simulink model "doa_no_gotos"  (R2013b)
settings: Solver=ode45  StartTime=0.0  StopTime=10.0  RelTol=1e-3
undefined symbols (not defined in the file or in its folder): calan_lib, comp_addsub
libraries: xbsIndex_r4 x1532, casper_library_misc x168, casper_library_delays x24
(part 2 of 16)

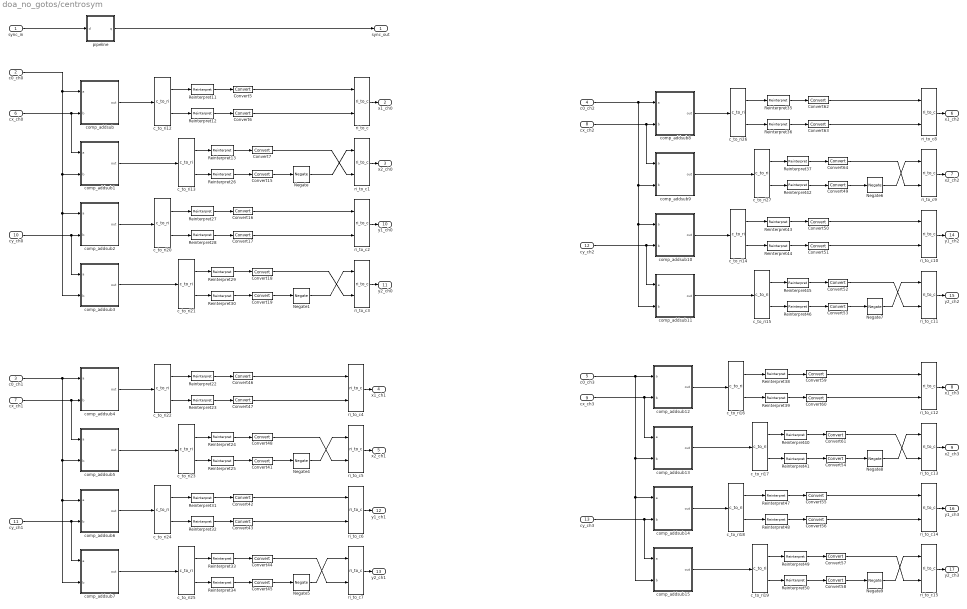
== system doa_no_gotos/centrosym ==
  sync_in : Inport
  c0_ch0 : Inport  Port=2
  c0_ch1 : Inport  Port=3
  c0_ch2 : Inport  Port=4
  c0_ch3 : Inport  Port=5
  cx_ch0 : Inport  Port=6
  cx_ch1 : Inport  Port=7
  cx_ch2 : Inport  Port=8
  cx_ch3 : Inport  Port=9
  cy_ch0 : Inport  Port=10
  cy_ch1 : Inport  Port=11
  cy_ch2 : Inport  Port=12
  cy_ch3 : Inport  Port=13
  Convert{5..7,15..19,41..64} (32 alike) : xbsIndex_r4/Convert  gui_display_data_type=Fixed-point  arith_type="Signed  (2's comp)"  n_bits=8  bin_pt=7  float_type=Single  exp_bits=8  fraction_bits=24  quantization="Round  (unbiased: +/- Inf)"  overflow=Saturate  en=off  latency=0  dbl_ovrd=off  pipeline=off  block_type=convert
  Negate{,1,4..9} (8 alike) : xbsIndex_r4/Negate  precision=User Defined  arith_type="Signed  (2's comp)"  n_bits=8  bin_pt=7  quantization="Round  (unbiased: +/- Inf)"  overflow=Saturate  en=off  latency=0  dbl_ovrd=off  block_type=negate
  Reinterpret{11..13,22..50} (32 alike) : xbsIndex_r4/Reinterpret  force_arith_type=on  arith_type="Signed  (2's comp)"  force_bin_pt=on  bin_pt=8  block_type=reinterpret
  c_to_ri{12..27} (16 alike) : casper_library_misc/c_to_ri  n_bits=9  bin_pt=7
      settings: AttributesFormatString=9_7 r/i
  comp_addsub : Subsystem  AncestorBlock=calan_lib/comp_addsub  mask(comp_addsub){addsub=Addition, n_bits_in=8, bin_pt_in=7, add_latency=2, n_bits_out=9, bin_pt_out=7, quantization=Round  (unbiased: +/- Inf), overflow=Saturate}
      mask prompts: addsub "Addition/Subtraction"; n_bits_in "Bit Width"; bin_pt_in "Binary Point"; add_latency "Adder Latency"; n_bits_out "Bit Width"; bin_pt_out "BInary Point"
      mask help: Add or substract two complex numbers of the same length.
      mask init:
      | comp_addsub_init(gcb, ...
      |     'addsub', addsub, ...
      |     'n_bits_in', n_bits_in, ...
      |     'bin_pt_in', bin_pt_in, ...
      |     'n_bits_out', n_bits_out, ...
      |     'bin_pt_out', bin_pt_out, ...
      |     'quantization', quantization, ...
      |     'overflow', overflow, ...
      |     'add_latency', add_latency);
      settings: AttributesFormatString=|
      | 8_7 * 8_7 ==> 9_7
      | Round  (unbiased: +/- Inf), Saturate
      mask TypeOptions addsub: Addition | Subtraction
      mask TypeOptions quantization: Truncate | Round  (unbiased: +/- Inf)
      mask TypeOptions overflow: Wrap | Saturate | Flag as error
      mask Display:
      | port_label('input', 1, 'a');
      | port_label('input', 2, 'b');
      | if strcmp(addsub, 'Addition')
      |     port_label('output', 1, 'a+b');
      | elseif strcmp(addsub, 'Subtraction')
      |     port_label('output', 1, 'a-b');
      | end
      | disp(['Z^-', num2str(add_latency)]);
  comp_addsub1 : Subsystem  AncestorBlock=calan_lib/comp_addsub  mask(comp_addsub){addsub=Subtraction, n_bits_in=8, bin_pt_in=7, add_latency=2, n_bits_out=9, bin_pt_out=7, quantization=Round  (unbiased: +/- Inf), overflow=Saturate}
      mask prompts: addsub "Addition/Subtraction"; n_bits_in "Bit Width"; bin_pt_in "Binary Point"; add_latency "Adder Latency"; n_bits_out "Bit Width"; bin_pt_out "BInary Point"
      mask help: Add or substract two complex numbers of the same length.
      mask init: same as doa_no_gotos/centrosym/comp_addsub
      settings: AttributesFormatString=|
      | 8_7 * 8_7 ==> 9_7
      | Round  (unbiased: +/- Inf), Saturate
      mask TypeOptions addsub: Addition | Subtraction
      mask TypeOptions quantization: Truncate | Round  (unbiased: +/- Inf)
      mask TypeOptions overflow: Wrap | Saturate | Flag as error
      mask Display:
      | port_label('input', 1, 'a');
      | port_label('input', 2, 'b');
      | if strcmp(addsub, 'Addition')
      |     port_label('output', 1, 'a+b');
      | elseif strcmp(addsub, 'Subtraction')
      |     port_label('output', 1, 'a-b');
      | end
      | disp(['Z^-', num2str(add_latency)]);
  comp_addsub10 : Subsystem  AncestorBlock=calan_lib/comp_addsub  mask(comp_addsub){addsub=Addition, n_bits_in=8, bin_pt_in=7, add_latency=2, n_bits_out=9, bin_pt_out=7, quantization=Round  (unbiased: +/- Inf), overflow=Saturate}
      mask prompts: addsub "Addition/Subtraction"; n_bits_in "Bit Width"; bin_pt_in "Binary Point"; add_latency "Adder Latency"; n_bits_out "Bit Width"; bin_pt_out "BInary Point"
      mask help: Add or substract two complex numbers of the same length.
      mask init: same as doa_no_gotos/centrosym/comp_addsub
      settings: AttributesFormatString=|
      | 8_7 * 8_7 ==> 9_7
      | Round  (unbiased: +/- Inf), Saturate
      mask TypeOptions addsub: Addition | Subtraction
      mask TypeOptions quantization: Truncate | Round  (unbiased: +/- Inf)
      mask TypeOptions overflow: Wrap | Saturate | Flag as error
      mask Display:
      | port_label('input', 1, 'a');
      | port_label('input', 2, 'b');
      | if strcmp(addsub, 'Addition')
      |     port_label('output', 1, 'a+b');
      | elseif strcmp(addsub, 'Subtraction')
      |     port_label('output', 1, 'a-b');
      | end
      | disp(['Z^-', num2str(add_latency)]);
  comp_addsub11 : Subsystem  AncestorBlock=calan_lib/comp_addsub  mask(comp_addsub){addsub=Subtraction, n_bits_in=8, bin_pt_in=7, add_latency=2, n_bits_out=9, bin_pt_out=7, quantization=Round  (unbiased: +/- Inf), overflow=Saturate}
      mask prompts: addsub "Addition/Subtraction"; n_bits_in "Bit Width"; bin_pt_in "Binary Point"; add_latency "Adder Latency"; n_bits_out "Bit Width"; bin_pt_out "BInary Point"
      mask help: Add or substract two complex numbers of the same length.
      mask init: same as doa_no_gotos/centrosym/comp_addsub
      settings: AttributesFormatString=|
      | 8_7 * 8_7 ==> 9_7
      | Round  (unbiased: +/- Inf), Saturate
      mask TypeOptions addsub: Addition | Subtraction
      mask TypeOptions quantization: Truncate | Round  (unbiased: +/- Inf)
      mask TypeOptions overflow: Wrap | Saturate | Flag as error
      mask Display:
      | port_label('input', 1, 'a');
      | port_label('input', 2, 'b');
      | if strcmp(addsub, 'Addition')
      |     port_label('output', 1, 'a+b');
      | elseif strcmp(addsub, 'Subtraction')
      |     port_label('output', 1, 'a-b');
      | end
      | disp(['Z^-', num2str(add_latency)]);
  comp_addsub12 : Subsystem  AncestorBlock=calan_lib/comp_addsub  mask(comp_addsub){addsub=Addition, n_bits_in=8, bin_pt_in=7, add_latency=2, n_bits_out=9, bin_pt_out=7, quantization=Round  (unbiased: +/- Inf), overflow=Saturate}
      mask prompts: addsub "Addition/Subtraction"; n_bits_in "Bit Width"; bin_pt_in "Binary Point"; add_latency "Adder Latency"; n_bits_out "Bit Width"; bin_pt_out "BInary Point"
      mask help: Add or substract two complex numbers of the same length.
      mask init: same as doa_no_gotos/centrosym/comp_addsub
      settings: AttributesFormatString=|
      | 8_7 * 8_7 ==> 9_7
      | Round  (unbiased: +/- Inf), Saturate
      mask TypeOptions addsub: Addition | Subtraction
      mask TypeOptions quantization: Truncate | Round  (unbiased: +/- Inf)
      mask TypeOptions overflow: Wrap | Saturate | Flag as error
      mask Display:
      | port_label('input', 1, 'a');
      | port_label('input', 2, 'b');
      | if strcmp(addsub, 'Addition')
      |     port_label('output', 1, 'a+b');
      | elseif strcmp(addsub, 'Subtraction')
      |     port_label('output', 1, 'a-b');
      | end
      | disp(['Z^-', num2str(add_latency)]);
  comp_addsub13 : Subsystem  AncestorBlock=calan_lib/comp_addsub  mask(comp_addsub){addsub=Subtraction, n_bits_in=8, bin_pt_in=7, add_latency=2, n_bits_out=9, bin_pt_out=7, quantization=Round  (unbiased: +/- Inf), overflow=Saturate}
      mask prompts: addsub "Addition/Subtraction"; n_bits_in "Bit Width"; bin_pt_in "Binary Point"; add_latency "Adder Latency"; n_bits_out "Bit Width"; bin_pt_out "BInary Point"
      mask help: Add or substract two complex numbers of the same length.
      mask init: same as doa_no_gotos/centrosym/comp_addsub
      settings: AttributesFormatString=|
      | 8_7 * 8_7 ==> 9_7
      | Round  (unbiased: +/- Inf), Saturate
      mask TypeOptions addsub: Addition | Subtraction
      mask TypeOptions quantization: Truncate | Round  (unbiased: +/- Inf)
      mask TypeOptions overflow: Wrap | Saturate | Flag as error
      mask Display:
      | port_label('input', 1, 'a');
      | port_label('input', 2, 'b');
      | if strcmp(addsub, 'Addition')
      |     port_label('output', 1, 'a+b');
      | elseif strcmp(addsub, 'Subtraction')
      |     port_label('output', 1, 'a-b');
      | end
      | disp(['Z^-', num2str(add_latency)]);
  comp_addsub14 : Subsystem  AncestorBlock=calan_lib/comp_addsub  mask(comp_addsub){addsub=Addition, n_bits_in=8, bin_pt_in=7, add_latency=2, n_bits_out=9, bin_pt_out=7, quantization=Round  (unbiased: +/- Inf), overflow=Saturate}
      mask prompts: addsub "Addition/Subtraction"; n_bits_in "Bit Width"; bin_pt_in "Binary Point"; add_latency "Adder Latency"; n_bits_out "Bit Width"; bin_pt_out "BInary Point"
      mask help: Add or substract two complex numbers of the same length.
      mask init: same as doa_no_gotos/centrosym/comp_addsub
      settings: AttributesFormatString=|
      | 8_7 * 8_7 ==> 9_7
      | Round  (unbiased: +/- Inf), Saturate
      mask TypeOptions addsub: Addition | Subtraction
      mask TypeOptions quantization: Truncate | Round  (unbiased: +/- Inf)
      mask TypeOptions overflow: Wrap | Saturate | Flag as error
      mask Display:
      | port_label('input', 1, 'a');
      | port_label('input', 2, 'b');
      | if strcmp(addsub, 'Addition')
      |     port_label('output', 1, 'a+b');
      | elseif strcmp(addsub, 'Subtraction')
      |     port_label('output', 1, 'a-b');
      | end
      | disp(['Z^-', num2str(add_latency)]);
  comp_addsub15 : Subsystem  AncestorBlock=calan_lib/comp_addsub  mask(comp_addsub){addsub=Subtraction, n_bits_in=8, bin_pt_in=7, add_latency=2, n_bits_out=9, bin_pt_out=7, quantization=Round  (unbiased: +/- Inf), overflow=Saturate}
      mask prompts: addsub "Addition/Subtraction"; n_bits_in "Bit Width"; bin_pt_in "Binary Point"; add_latency "Adder Latency"; n_bits_out "Bit Width"; bin_pt_out "BInary Point"
      mask help: Add or substract two complex numbers of the same length.
      mask init: same as doa_no_gotos/centrosym/comp_addsub
      settings: AttributesFormatString=|
      | 8_7 * 8_7 ==> 9_7
      | Round  (unbiased: +/- Inf), Saturate
      mask TypeOptions addsub: Addition | Subtraction
      mask TypeOptions quantization: Truncate | Round  (unbiased: +/- Inf)
      mask TypeOptions overflow: Wrap | Saturate | Flag as error
      mask Display:
      | port_label('input', 1, 'a');
      | port_label('input', 2, 'b');
      | if strcmp(addsub, 'Addition')
      |     port_label('output', 1, 'a+b');
      | elseif strcmp(addsub, 'Subtraction')
      |     port_label('output', 1, 'a-b');
      | end
      | disp(['Z^-', num2str(add_latency)]);
  comp_addsub2 : Subsystem  AncestorBlock=calan_lib/comp_addsub  mask(comp_addsub){addsub=Addition, n_bits_in=8, bin_pt_in=7, add_latency=2, n_bits_out=9, bin_pt_out=7, quantization=Round  (unbiased: +/- Inf), overflow=Saturate}
      mask prompts: addsub "Addition/Subtraction"; n_bits_in "Bit Width"; bin_pt_in "Binary Point"; add_latency "Adder Latency"; n_bits_out "Bit Width"; bin_pt_out "BInary Point"
      mask help: Add or substract two complex numbers of the same length.
      mask init: same as doa_no_gotos/centrosym/comp_addsub
      settings: AttributesFormatString=|
      | 8_7 * 8_7 ==> 9_7
      | Round  (unbiased: +/- Inf), Saturate
      mask TypeOptions addsub: Addition | Subtraction
      mask TypeOptions quantization: Truncate | Round  (unbiased: +/- Inf)
      mask TypeOptions overflow: Wrap | Saturate | Flag as error
      mask Display:
      | port_label('input', 1, 'a');
      | port_label('input', 2, 'b');
      | if strcmp(addsub, 'Addition')
      |     port_label('output', 1, 'a+b');
      | elseif strcmp(addsub, 'Subtraction')
      |     port_label('output', 1, 'a-b');
      | end
      | disp(['Z^-', num2str(add_latency)]);
  comp_addsub3 : Subsystem  AncestorBlock=calan_lib/comp_addsub  mask(comp_addsub){addsub=Subtraction, n_bits_in=8, bin_pt_in=7, add_latency=2, n_bits_out=9, bin_pt_out=7, quantization=Round  (unbiased: +/- Inf), overflow=Saturate}
      mask prompts: addsub "Addition/Subtraction"; n_bits_in "Bit Width"; bin_pt_in "Binary Point"; add_latency "Adder Latency"; n_bits_out "Bit Width"; bin_pt_out "BInary Point"
      mask help: Add or substract two complex numbers of the same length.
      mask init: same as doa_no_gotos/centrosym/comp_addsub
      settings: AttributesFormatString=|
      | 8_7 * 8_7 ==> 9_7
      | Round  (unbiased: +/- Inf), Saturate
      mask TypeOptions addsub: Addition | Subtraction
      mask TypeOptions quantization: Truncate | Round  (unbiased: +/- Inf)
      mask TypeOptions overflow: Wrap | Saturate | Flag as error
      mask Display:
      | port_label('input', 1, 'a');
      | port_label('input', 2, 'b');
      | if strcmp(addsub, 'Addition')
      |     port_label('output', 1, 'a+b');
      | elseif strcmp(addsub, 'Subtraction')
      |     port_label('output', 1, 'a-b');
      | end
      | disp(['Z^-', num2str(add_latency)]);
  comp_addsub4 : Subsystem  AncestorBlock=calan_lib/comp_addsub  mask(comp_addsub){addsub=Addition, n_bits_in=8, bin_pt_in=7, add_latency=2, n_bits_out=9, bin_pt_out=7, quantization=Round  (unbiased: +/- Inf), overflow=Saturate}
      mask prompts: addsub "Addition/Subtraction"; n_bits_in "Bit Width"; bin_pt_in "Binary Point"; add_latency "Adder Latency"; n_bits_out "Bit Width"; bin_pt_out "BInary Point"
      mask help: Add or substract two complex numbers of the same length.
      mask init: same as doa_no_gotos/centrosym/comp_addsub
      settings: AttributesFormatString=|
      | 8_7 * 8_7 ==> 9_7
      | Round  (unbiased: +/- Inf), Saturate
      mask TypeOptions addsub: Addition | Subtraction
      mask TypeOptions quantization: Truncate | Round  (unbiased: +/- Inf)
      mask TypeOptions overflow: Wrap | Saturate | Flag as error
      mask Display:
      | port_label('input', 1, 'a');
      | port_label('input', 2, 'b');
      | if strcmp(addsub, 'Addition')
      |     port_label('output', 1, 'a+b');
      | elseif strcmp(addsub, 'Subtraction')
      |     port_label('output', 1, 'a-b');
      | end
      | disp(['Z^-', num2str(add_latency)]);
  comp_addsub5 : Subsystem  AncestorBlock=calan_lib/comp_addsub  mask(comp_addsub){addsub=Subtraction, n_bits_in=8, bin_pt_in=7, add_latency=2, n_bits_out=9, bin_pt_out=7, quantization=Round  (unbiased: +/- Inf), overflow=Saturate}
      mask prompts: addsub "Addition/Subtraction"; n_bits_in "Bit Width"; bin_pt_in "Binary Point"; add_latency "Adder Latency"; n_bits_out "Bit Width"; bin_pt_out "BInary Point"
      mask help: Add or substract two complex numbers of the same length.
      mask init: same as doa_no_gotos/centrosym/comp_addsub
      settings: AttributesFormatString=|
      | 8_7 * 8_7 ==> 9_7
      | Round  (unbiased: +/- Inf), Saturate
      mask TypeOptions addsub: Addition | Subtraction
      mask TypeOptions quantization: Truncate | Round  (unbiased: +/- Inf)
      mask TypeOptions overflow: Wrap | Saturate | Flag as error
      mask Display:
      | port_label('input', 1, 'a');
      | port_label('input', 2, 'b');
      | if strcmp(addsub, 'Addition')
      |     port_label('output', 1, 'a+b');
      | elseif strcmp(addsub, 'Subtraction')
      |     port_label('output', 1, 'a-b');
      | end
      | disp(['Z^-', num2str(add_latency)]);
  comp_addsub6 : Subsystem  AncestorBlock=calan_lib/comp_addsub  mask(comp_addsub){addsub=Addition, n_bits_in=8, bin_pt_in=7, add_latency=2, n_bits_out=9, bin_pt_out=7, quantization=Round  (unbiased: +/- Inf), overflow=Saturate}
      mask prompts: addsub "Addition/Subtraction"; n_bits_in "Bit Width"; bin_pt_in "Binary Point"; add_latency "Adder Latency"; n_bits_out "Bit Width"; bin_pt_out "BInary Point"
      mask help: Add or substract two complex numbers of the same length.
      mask init: same as doa_no_gotos/centrosym/comp_addsub
      settings: AttributesFormatString=|
      | 8_7 * 8_7 ==> 9_7
      | Round  (unbiased: +/- Inf), Saturate
      mask TypeOptions addsub: Addition | Subtraction
      mask TypeOptions quantization: Truncate | Round  (unbiased: +/- Inf)
      mask TypeOptions overflow: Wrap | Saturate | Flag as error
      mask Display:
      | port_label('input', 1, 'a');
      | port_label('input', 2, 'b');
      | if strcmp(addsub, 'Addition')
      |     port_label('output', 1, 'a+b');
      | elseif strcmp(addsub, 'Subtraction')
      |     port_label('output', 1, 'a-b');
      | end
      | disp(['Z^-', num2str(add_latency)]);
  comp_addsub7 : Subsystem  AncestorBlock=calan_lib/comp_addsub  mask(comp_addsub){addsub=Subtraction, n_bits_in=8, bin_pt_in=7, add_latency=2, n_bits_out=9, bin_pt_out=7, quantization=Round  (unbiased: +/- Inf), overflow=Saturate}
      mask prompts: addsub "Addition/Subtraction"; n_bits_in "Bit Width"; bin_pt_in "Binary Point"; add_latency "Adder Latency"; n_bits_out "Bit Width"; bin_pt_out "BInary Point"
      mask help: Add or substract two complex numbers of the same length.
      mask init: same as doa_no_gotos/centrosym/comp_addsub
      settings: AttributesFormatString=|
      | 8_7 * 8_7 ==> 9_7
      | Round  (unbiased: +/- Inf), Saturate
      mask TypeOptions addsub: Addition | Subtraction
      mask TypeOptions quantization: Truncate | Round  (unbiased: +/- Inf)
      mask TypeOptions overflow: Wrap | Saturate | Flag as error
      mask Display:
      | port_label('input', 1, 'a');
      | port_label('input', 2, 'b');
      | if strcmp(addsub, 'Addition')
      |     port_label('output', 1, 'a+b');
      | elseif strcmp(addsub, 'Subtraction')
      |     port_label('output', 1, 'a-b');
      | end
      | disp(['Z^-', num2str(add_latency)]);
  comp_addsub8 : Subsystem  AncestorBlock=calan_lib/comp_addsub  mask(comp_addsub){addsub=Addition, n_bits_in=8, bin_pt_in=7, add_latency=2, n_bits_out=9, bin_pt_out=7, quantization=Round  (unbiased: +/- Inf), overflow=Saturate}
      mask prompts: addsub "Addition/Subtraction"; n_bits_in "Bit Width"; bin_pt_in "Binary Point"; add_latency "Adder Latency"; n_bits_out "Bit Width"; bin_pt_out "BInary Point"
      mask help: Add or substract two complex numbers of the same length.
      mask init: same as doa_no_gotos/centrosym/comp_addsub
      settings: AttributesFormatString=|
      | 8_7 * 8_7 ==> 9_7
      | Round  (unbiased: +/- Inf), Saturate
      mask TypeOptions addsub: Addition | Subtraction
      mask TypeOptions quantization: Truncate | Round  (unbiased: +/- Inf)
      mask TypeOptions overflow: Wrap | Saturate | Flag as error
      mask Display:
      | port_label('input', 1, 'a');
      | port_label('input', 2, 'b');
      | if strcmp(addsub, 'Addition')
      |     port_label('output', 1, 'a+b');
      | elseif strcmp(addsub, 'Subtraction')
      |     port_label('output', 1, 'a-b');
      | end
      | disp(['Z^-', num2str(add_latency)]);
  comp_addsub9 : Subsystem  AncestorBlock=calan_lib/comp_addsub  mask(comp_addsub){addsub=Subtraction, n_bits_in=8, bin_pt_in=7, add_latency=2, n_bits_out=9, bin_pt_out=7, quantization=Round  (unbiased: +/- Inf), overflow=Saturate}
      mask prompts: addsub "Addition/Subtraction"; n_bits_in "Bit Width"; bin_pt_in "Binary Point"; add_latency "Adder Latency"; n_bits_out "Bit Width"; bin_pt_out "BInary Point"
      mask help: Add or substract two complex numbers of the same length.
      mask init: same as doa_no_gotos/centrosym/comp_addsub
      settings: AttributesFormatString=|
      | 8_7 * 8_7 ==> 9_7
      | Round  (unbiased: +/- Inf), Saturate
      mask TypeOptions addsub: Addition | Subtraction
      mask TypeOptions quantization: Truncate | Round  (unbiased: +/- Inf)
      mask TypeOptions overflow: Wrap | Saturate | Flag as error
      mask Display:
      | port_label('input', 1, 'a');
      | port_label('input', 2, 'b');
      | if strcmp(addsub, 'Addition')
      |     port_label('output', 1, 'a+b');
      | elseif strcmp(addsub, 'Subtraction')
      |     port_label('output', 1, 'a-b');
      | end
      | disp(['Z^-', num2str(add_latency)]);
  pipeline : Subsystem  AncestorBlock=casper_library_delays/pipeline  mask(pipeline){latency=2}
      mask help:
      | An explicitly laid-out delay line to avoid mapping to SRL16s
      | for use in pipelining to help achieve timing closure.
      mask init:
      | pipeline_init(gcb,'latency',latency);
      settings: AttributesFormatString=Latency = %<latency>
      mask Display:
      | port_label('input', 1, 'd');
      | port_label('output', 1, 'q');
      | disp(['Z^-', num2str(latency)]);
  ri_to_c{,1..15} (16 alike) : casper_library_misc/ri_to_c
  sync_out : Outport
  x1_ch0 : Outport  Port=2
  x2_ch0 : Outport  Port=3
  x1_ch1 : Outport  Port=4
  x2_ch1 : Outport  Port=5
  x1_ch2 : Outport  Port=6
  x2_ch2 : Outport  Port=7
  x1_ch3 : Outport  Port=8
  x2_ch3 : Outport  Port=9
  y1_ch0 : Outport  Port=10
  y2_ch0 : Outport  Port=11
  y1_ch1 : Outport  Port=12
  y2_ch1 : Outport  Port=13
  y1_ch2 : Outport  Port=14
  y2_ch2 : Outport  Port=15
  y1_ch3 : Outport  Port=16
  y2_ch3 : Outport  Port=17
  wires:
  c0_ch0/1 -> comp_addsub/1(a), comp_addsub3/2(b), comp_addsub2/1(a), comp_addsub1/2(b)
  cy_ch0/1 -> comp_addsub3/1(a), comp_addsub2/2(b)
  comp_addsub/1(out) -> c_to_ri12/1
  c_to_ri12/1 -> Reinterpret11/1
  c_to_ri12/2 -> Reinterpret12/1
  comp_addsub1/1(out) -> c_to_ri13/1
  comp_addsub2/1(out) -> c_to_ri20/1
  comp_addsub3/1(out) -> c_to_ri21/1
  c_to_ri13/1 -> Reinterpret13/1
  c_to_ri13/2 -> Reinterpret26/1
  c_to_ri20/1 -> Reinterpret27/1
  c_to_ri20/2 -> Reinterpret28/1
  c_to_ri21/1 -> Reinterpret29/1
  c_to_ri21/2 -> Reinterpret30/1
  Convert7/1 -> ri_to_c1/2
  Convert18/1 -> ri_to_c3/2
  cx_ch0/1 -> comp_addsub/2(b), comp_addsub1/1(a)
  Reinterpret11/1 -> Convert5/1
  Reinterpret12/1 -> Convert6/1
  Reinterpret13/1 -> Convert7/1
  Convert15/1 -> Negate/1
  Reinterpret26/1 -> Convert15/1
  Reinterpret27/1 -> Convert16/1
  Convert16/1 -> ri_to_c2/1
  Reinterpret28/1 -> Convert17/1
  Convert17/1 -> ri_to_c2/2
  Reinterpret29/1 -> Convert18/1
  Convert19/1 -> Negate1/1
  Reinterpret30/1 -> Convert19/1
  Negate/1 -> ri_to_c1/1
  Negate1/1 -> ri_to_c3/1
  c0_ch2/1 -> comp_addsub10/1(a), comp_addsub11/2(b), comp_addsub9/2(b), comp_addsub8/1(a)
  cy_ch2/1 -> comp_addsub10/2(b), comp_addsub11/1(a)
  comp_addsub8/1(out) -> c_to_ri26/1
  c_to_ri26/1 -> Reinterpret35/1
  c_to_ri26/2 -> Reinterpret36/1
  comp_addsub9/1(out) -> c_to_ri27/1
  comp_addsub10/1(out) -> c_to_ri14/1
  comp_addsub11/1(out) -> c_to_ri15/1
  c_to_ri27/1 -> Reinterpret37/1
  c_to_ri27/2 -> Reinterpret42/1
  c_to_ri14/1 -> Reinterpret43/1
  c_to_ri14/2 -> Reinterpret44/1
  c_to_ri15/1 -> Reinterpret45/1
  c_to_ri15/2 -> Reinterpret46/1
  cx_ch2/1 -> comp_addsub9/1(a), comp_addsub8/2(b)
  Reinterpret35/1 -> Convert62/1
  Reinterpret36/1 -> Convert63/1
  Reinterpret37/1 -> Convert64/1
  Convert49/1 -> Negate6/1
  Reinterpret42/1 -> Convert49/1
  Reinterpret43/1 -> Convert50/1
  Reinterpret44/1 -> Convert51/1
  Reinterpret45/1 -> Convert52/1
  Convert53/1 -> Negate7/1
  Reinterpret46/1 -> Convert53/1
  c0_ch1/1 -> comp_addsub6/1(a), comp_addsub7/2(b), comp_addsub5/2(b), comp_addsub4/1(a)
  cy_ch1/1 -> comp_addsub6/2(b), comp_addsub7/1(a)
  comp_addsub4/1(out) -> c_to_ri22/1
  c_to_ri22/1 -> Reinterpret22/1
  c_to_ri22/2 -> Reinterpret23/1
  comp_addsub5/1(out) -> c_to_ri23/1
  comp_addsub6/1(out) -> c_to_ri24/1
  comp_addsub7/1(out) -> c_to_ri25/1
  c_to_ri23/1 -> Reinterpret24/1
  c_to_ri23/2 -> Reinterpret25/1
  c_to_ri24/1 -> Reinterpret31/1
  c_to_ri24/2 -> Reinterpret32/1
  c_to_ri25/1 -> Reinterpret33/1
  c_to_ri25/2 -> Reinterpret34/1
  cx_ch1/1 -> comp_addsub5/1(a), comp_addsub4/2(b)
  Reinterpret22/1 -> Convert46/1
  Reinterpret23/1 -> Convert47/1
  Reinterpret24/1 -> Convert48/1
  Convert41/1 -> Negate4/1
  Reinterpret25/1 -> Convert41/1
  Reinterpret31/1 -> Convert42/1
  Reinterpret32/1 -> Convert43/1
  Reinterpret33/1 -> Convert44/1
  Convert45/1 -> Negate5/1
  Reinterpret34/1 -> Convert45/1
  c0_ch3/1 -> comp_addsub12/1(a), comp_addsub15/2(b), comp_addsub14/1(a), comp_addsub13/2(b)
  cy_ch3/1 -> comp_addsub15/1(a), comp_addsub14/2(b)
  comp_addsub12/1(out) -> c_to_ri16/1
  c_to_ri16/1 -> Reinterpret38/1
  c_to_ri16/2 -> Reinterpret39/1
  comp_addsub13/1(out) -> c_to_ri17/1
  comp_addsub14/1(out) -> c_to_ri18/1
  comp_addsub15/1(out) -> c_to_ri19/1
  c_to_ri17/1 -> Reinterpret40/1
  c_to_ri17/2 -> Reinterpret41/1
  c_to_ri18/1 -> Reinterpret47/1
  c_to_ri18/2 -> Reinterpret48/1
  c_to_ri19/1 -> Reinterpret49/1
  c_to_ri19/2 -> Reinterpret50/1
  cx_ch3/1 -> comp_addsub12/2(b), comp_addsub13/1(a)
  Reinterpret38/1 -> Convert59/1
  Reinterpret39/1 -> Convert60/1
  Reinterpret40/1 -> Convert61/1
  Convert54/1 -> Negate8/1
  Reinterpret41/1 -> Convert54/1
  Reinterpret47/1 -> Convert55/1
  Reinterpret48/1 -> Convert56/1
  Reinterpret49/1 -> Convert57/1
  Convert58/1 -> Negate9/1
  Reinterpret50/1 -> Convert58/1
  Convert5/1 -> ri_to_c/1
  Convert6/1 -> ri_to_c/2
  ri_to_c/1 -> x1_ch0/1
  ri_to_c1/1 -> x2_ch0/1
  ri_to_c2/1 -> y1_ch0/1
  ri_to_c3/1 -> y2_ch0/1
  ri_to_c4/1 -> x1_ch1/1
  Convert46/1 -> ri_to_c4/1
  Convert47/1 -> ri_to_c4/2
  ri_to_c5/1 -> x2_ch1/1
  Negate4/1 -> ri_to_c5/1
  Convert48/1 -> ri_to_c5/2
  ri_to_c6/1 -> y1_ch1/1
  Convert42/1 -> ri_to_c6/1
  Convert43/1 -> ri_to_c6/2
  ri_to_c7/1 -> y2_ch1/1
  Negate5/1 -> ri_to_c7/1
  Convert44/1 -> ri_to_c7/2
  ri_to_c8/1 -> x1_ch2/1
  Convert62/1 -> ri_to_c8/1
  Convert63/1 -> ri_to_c8/2
  ri_to_c9/1 -> x2_ch2/1
  Negate6/1 -> ri_to_c9/1
  Convert64/1 -> ri_to_c9/2
  ri_to_c10/1 -> y1_ch2/1
  Convert50/1 -> ri_to_c10/1
  Convert51/1 -> ri_to_c10/2
  ri_to_c11/1 -> y2_ch2/1
  Negate7/1 -> ri_to_c11/1
  Convert52/1 -> ri_to_c11/2
  ri_to_c12/1 -> x1_ch3/1
  Convert59/1 -> ri_to_c12/1
  Convert60/1 -> ri_to_c12/2
  ri_to_c13/1 -> x2_ch3/1
  Negate8/1 -> ri_to_c13/1
  Convert61/1 -> ri_to_c13/2
  ri_to_c14/1 -> y1_ch3/1
  Convert55/1 -> ri_to_c14/1
  Convert56/1 -> ri_to_c14/2
  ri_to_c15/1 -> y2_ch3/1
  Negate9/1 -> ri_to_c15/1
  Convert57/1 -> ri_to_c15/2
  sync_in/1 -> pipeline/1(d)
  pipeline/1(q) -> sync_out/1

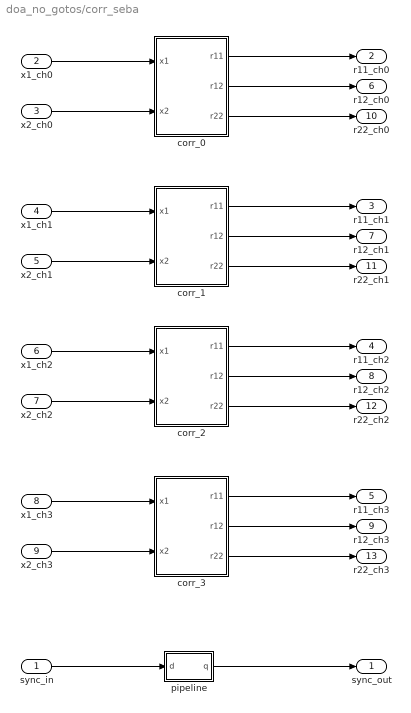
== system doa_no_gotos/corr_seba ==
  sync_in : Inport
  x1_ch0 : Inport  Port=2
  x2_ch0 : Inport  Port=3
  x1_ch1 : Inport  Port=4
  x2_ch1 : Inport  Port=5
  x1_ch2 : Inport  Port=6
  x2_ch2 : Inport  Port=7
  x1_ch3 : Inport  Port=8
  x2_ch3 : Inport  Port=9
  corr_0 : Subsystem
  corr_1 : Subsystem
  corr_2 : Subsystem
  corr_3 : Subsystem
  pipeline : Subsystem  AncestorBlock=casper_library_delays/pipeline  mask(pipeline){latency=7}
      mask help:
      | An explicitly laid-out delay line to avoid mapping to SRL16s
      | for use in pipelining to help achieve timing closure.
      mask init:
      | pipeline_init(gcb,'latency',latency);
      settings: AttributesFormatString=Latency = %<latency>
      mask Display:
      | port_label('input', 1, 'd');
      | port_label('output', 1, 'q');
      | disp(['Z^-', num2str(latency)]);
  sync_out : Outport
  r11_ch0 : Outport  Port=2
  r11_ch1 : Outport  Port=3
  r11_ch2 : Outport  Port=4
  r11_ch3 : Outport  Port=5
  r12_ch0 : Outport  Port=6
  r12_ch1 : Outport  Port=7
  r12_ch2 : Outport  Port=8
  r12_ch3 : Outport  Port=9
  r22_ch0 : Outport  Port=10
  r22_ch1 : Outport  Port=11
  r22_ch2 : Outport  Port=12
  r22_ch3 : Outport  Port=13
  wires:
  corr_0/2(r12) -> r12_ch0/1
  corr_0/3(r22) -> r22_ch0/1
  x1_ch0/1 -> corr_0/1(x1)
  x2_ch0/1 -> corr_0/2(x2)
  corr_0/1(r11) -> r11_ch0/1
  corr_1/2(r12) -> r12_ch1/1
  corr_1/3(r22) -> r22_ch1/1
  x1_ch1/1 -> corr_1/1(x1)
  x2_ch1/1 -> corr_1/2(x2)
  corr_1/1(r11) -> r11_ch1/1
  corr_2/2(r12) -> r12_ch2/1
  corr_2/3(r22) -> r22_ch2/1
  x1_ch2/1 -> corr_2/1(x1)
  x2_ch2/1 -> corr_2/2(x2)
  corr_2/1(r11) -> r11_ch2/1
  corr_3/2(r12) -> r12_ch3/1
  corr_3/3(r22) -> r22_ch3/1
  x1_ch3/1 -> corr_3/1(x1)
  x2_ch3/1 -> corr_3/2(x2)
  corr_3/1(r11) -> r11_ch3/1
  sync_in/1 -> pipeline/1(d)
  pipeline/1(q) -> sync_out/1

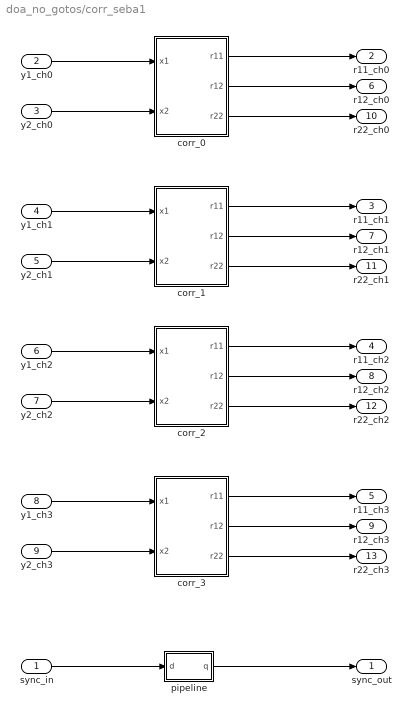
== system doa_no_gotos/corr_seba1 ==
  sync_in : Inport
  y1_ch0 : Inport  Port=2
  y2_ch0 : Inport  Port=3
  y1_ch1 : Inport  Port=4
  y2_ch1 : Inport  Port=5
  y1_ch2 : Inport  Port=6
  y2_ch2 : Inport  Port=7
  y1_ch3 : Inport  Port=8
  y2_ch3 : Inport  Port=9
  corr_0 : Subsystem
  corr_1 : Subsystem
  corr_2 : Subsystem
  corr_3 : Subsystem
  pipeline : Subsystem  AncestorBlock=casper_library_delays/pipeline  mask(pipeline){latency=7}
      mask help:
      | An explicitly laid-out delay line to avoid mapping to SRL16s
      | for use in pipelining to help achieve timing closure.
      mask init:
      | pipeline_init(gcb,'latency',latency);
      settings: AttributesFormatString=Latency = %<latency>
      mask Display:
      | port_label('input', 1, 'd');
      | port_label('output', 1, 'q');
      | disp(['Z^-', num2str(latency)]);
  sync_out : Outport
  r11_ch0 : Outport  Port=2
  r11_ch1 : Outport  Port=3
  r11_ch2 : Outport  Port=4
  r11_ch3 : Outport  Port=5
  r12_ch0 : Outport  Port=6
  r12_ch1 : Outport  Port=7
  r12_ch2 : Outport  Port=8
  r12_ch3 : Outport  Port=9
  r22_ch0 : Outport  Port=10
  r22_ch1 : Outport  Port=11
  r22_ch2 : Outport  Port=12
  r22_ch3 : Outport  Port=13
  wires:
  corr_0/2(r12) -> r12_ch0/1
  corr_0/3(r22) -> r22_ch0/1
  y1_ch0/1 -> corr_0/1(x1)
  y2_ch0/1 -> corr_0/2(x2)
  corr_0/1(r11) -> r11_ch0/1
  corr_1/2(r12) -> r12_ch1/1
  corr_1/3(r22) -> r22_ch1/1
  y1_ch1/1 -> corr_1/1(x1)
  y2_ch1/1 -> corr_1/2(x2)
  corr_1/1(r11) -> r11_ch1/1
  corr_2/2(r12) -> r12_ch2/1
  corr_2/3(r22) -> r22_ch2/1
  y1_ch2/1 -> corr_2/1(x1)
  y2_ch2/1 -> corr_2/2(x2)
  corr_2/1(r11) -> r11_ch2/1
  corr_3/2(r12) -> r12_ch3/1
  corr_3/3(r22) -> r22_ch3/1
  y1_ch3/1 -> corr_3/1(x1)
  y2_ch3/1 -> corr_3/2(x2)
  corr_3/1(r11) -> r11_ch3/1
  sync_in/1 -> pipeline/1(d)
  pipeline/1(q) -> sync_out/1

== system doa_no_gotos/edge_detect ==
  in : Inport
  Delay : xbsIndex_r4/Delay  rst=off  infoeditControl=Selection of Reset will increase slice count due to use of real FFs and instead of SRLs  en=off  latency=1  dbl_ovrd=off  reg_retiming=on  block_type=delay
      settings: xl_area=[0, 0, 0, 0, 0, 0, 0]
  Inverter : xbsIndex_r4/Inverter  en=off  latency=0  dbl_ovrd=off  block_type=inv
      settings: xl_area=[0, 0, 0, 0, 0, 0, 0]
  edge_op : xbsIndex_r4/Logical  logical_function=AND  inputs=2  en=off  latency=0  precision=Full  arith_type=Unsigned  n_bits=8  bin_pt=2  align_bp=on  dbl_ovrd=off  block_type=logical
      settings: xl_area=[0, 0, 0, 0, 0, 0, 0]
  out : Outport
  wires:
  Inverter/1 -> edge_op/1
  edge_op/1 -> out/1
  in/1 -> Inverter/1, Delay/1
  Delay/1 -> edge_op/2

== system doa_no_gotos/edge_detect1 ==
  in : Inport
  Delay : xbsIndex_r4/Delay  rst=off  infoeditControl=Selection of Reset will increase slice count due to use of real FFs and instead of SRLs  en=off  latency=1  dbl_ovrd=off  reg_retiming=on  block_type=delay
      settings: xl_area=[0, 0, 0, 0, 0, 0, 0]
  Inverter : xbsIndex_r4/Inverter  en=off  latency=0  dbl_ovrd=off  block_type=inv
      settings: xl_area=[0, 0, 0, 0, 0, 0, 0]
  edge_op : xbsIndex_r4/Logical  logical_function=AND  inputs=2  en=off  latency=0  precision=Full  arith_type=Unsigned  n_bits=8  bin_pt=2  align_bp=on  dbl_ovrd=off  block_type=logical
      settings: xl_area=[0, 0, 0, 0, 0, 0, 0]
  out : Outport
  wires:
  Inverter/1 -> edge_op/1
  edge_op/1 -> out/1
  in/1 -> Inverter/1, Delay/1
  Delay/1 -> edge_op/2

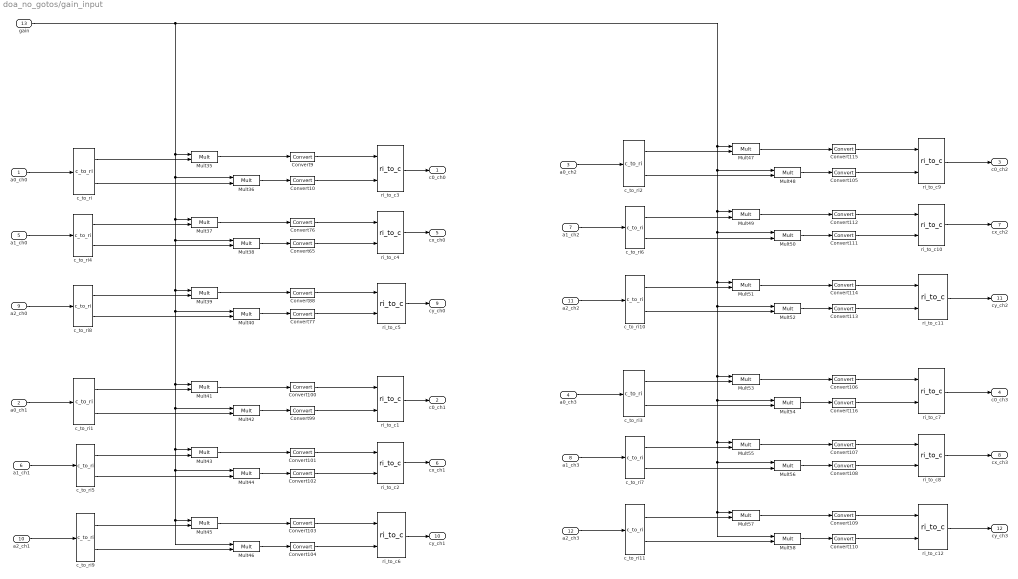
== system doa_no_gotos/gain_input ==
  a0_ch0 : Inport
  a0_ch1 : Inport  Port=2
  a0_ch2 : Inport  Port=3
  a0_ch3 : Inport  Port=4
  a1_ch0 : Inport  Port=5
  a1_ch1 : Inport  Port=6
  a1_ch2 : Inport  Port=7
  a1_ch3 : Inport  Port=8
  a2_ch0 : Inport  Port=9
  a2_ch1 : Inport  Port=10
  a2_ch2 : Inport  Port=11
  a2_ch3 : Inport  Port=12
  gain : Inport  Port=13
  Convert{9..10,65,76..77,88,99..116} (24 alike) : xbsIndex_r4/Convert  gui_display_data_type=Fixed-point  arith_type="Signed  (2's comp)"  n_bits=8  bin_pt=7  float_type=Single  exp_bits=8  fraction_bits=24  quantization="Round  (unbiased: +/- Inf)"  overflow=Saturate  en=off  latency=0  dbl_ovrd=off  pipeline=off  block_type=convert
  Mult{35..58} (24 alike) : xbsIndex_r4/Mult  precision=Full  arith_type="Signed  (2's comp)"  n_bits=16  bin_pt=14  quantization=Truncate  overflow=Wrap  en=off  latency=3  dbl_ovrd=off  use_behavioral_HDL=off  opt=Speed  use_embedded=on  optimum_pipeline=off  pipeline=on  use_rpm=on  placement_style=Triangular  block_type=mult
  c_to_ri{,1..11} (12 alike) : casper_library_misc/c_to_ri  n_bits=18  bin_pt=17
  ri_to_c{1..12} (12 alike) : casper_library_misc/ri_to_c
  c0_ch0 : Outport
  c0_ch1 : Outport  Port=2
  c0_ch2 : Outport  Port=3
  c0_ch3 : Outport  Port=4
  cx_ch0 : Outport  Port=5
  cx_ch1 : Outport  Port=6
  cx_ch2 : Outport  Port=7
  cx_ch3 : Outport  Port=8
  cy_ch0 : Outport  Port=9
  cy_ch1 : Outport  Port=10
  cy_ch2 : Outport  Port=11
  cy_ch3 : Outport  Port=12
  wires:
  c_to_ri/1 -> Mult35/2
  c_to_ri/2 -> Mult36/2
  Mult35/1 -> Convert9/1
  Mult36/1 -> Convert10/1
  Convert10/1 -> ri_to_c3/2
  Convert9/1 -> ri_to_c3/1
  c_to_ri4/1 -> Mult37/2
  c_to_ri4/2 -> Mult38/2
  c_to_ri8/1 -> Mult39/2
  c_to_ri8/2 -> Mult40/2
  c_to_ri1/1 -> Mult41/2
  c_to_ri1/2 -> Mult42/2
  c_to_ri5/1 -> Mult43/2
  c_to_ri5/2 -> Mult44/2
  c_to_ri9/1 -> Mult45/2
  c_to_ri9/2 -> Mult46/2
  Mult37/1 -> Convert76/1
  Convert76/1 -> ri_to_c4/1
  Mult38/1 -> Convert65/1
  Convert65/1 -> ri_to_c4/2
  Mult39/1 -> Convert88/1
  Convert88/1 -> ri_to_c5/1
  Mult40/1 -> Convert77/1
  Convert77/1 -> ri_to_c5/2
  Mult41/1 -> Convert100/1
  Convert100/1 -> ri_to_c1/1
  Mult42/1 -> Convert99/1
  Convert99/1 -> ri_to_c1/2
  Mult43/1 -> Convert101/1
  Convert101/1 -> ri_to_c2/1
  Mult44/1 -> Convert102/1
  Convert102/1 -> ri_to_c2/2
  Convert103/1 -> ri_to_c6/1
  Mult45/1 -> Convert103/1
  Mult46/1 -> Convert104/1
  Convert104/1 -> ri_to_c6/2
  gain/1 -> Mult46/1, Mult45/1, Mult44/1, Mult43/1, Mult42/1, Mult41/1, Mult40/1, Mult39/1, Mult38/1, Mult37/1, Mult36/1, Mult35/1, Mult47/1, Mult48/1, Mult49/1, Mult50/1, Mult51/1, Mult52/1, Mult53/1, Mult54/1, Mult55/1, Mult56/1, Mult57/1, Mult58/1
  c_to_ri2/1 -> Mult47/2
  c_to_ri2/2 -> Mult48/2
  Mult47/1 -> Convert115/1
  Mult48/1 -> Convert105/1
  Convert105/1 -> ri_to_c9/2
  Convert115/1 -> ri_to_c9/1
  c_to_ri6/1 -> Mult49/2
  c_to_ri6/2 -> Mult50/2
  c_to_ri10/1 -> Mult51/2
  c_to_ri10/2 -> Mult52/2
  c_to_ri3/1 -> Mult53/2
  c_to_ri3/2 -> Mult54/2
  c_to_ri7/1 -> Mult55/2
  c_to_ri7/2 -> Mult56/2
  c_to_ri11/1 -> Mult57/2
  c_to_ri11/2 -> Mult58/2
  Mult49/1 -> Convert112/1
  Convert112/1 -> ri_to_c10/1
  Mult50/1 -> Convert111/1
  Convert111/1 -> ri_to_c10/2
  Mult51/1 -> Convert114/1
  Convert114/1 -> ri_to_c11/1
  Mult52/1 -> Convert113/1
  Convert113/1 -> ri_to_c11/2
  Mult53/1 -> Convert106/1
  Convert106/1 -> ri_to_c7/1
  Mult54/1 -> Convert116/1
  Convert116/1 -> ri_to_c7/2
  Mult55/1 -> Convert107/1
  Convert107/1 -> ri_to_c8/1
  Mult56/1 -> Convert108/1
  Convert108/1 -> ri_to_c8/2
  Convert109/1 -> ri_to_c12/1
  Mult57/1 -> Convert109/1
  Mult58/1 -> Convert110/1
  Convert110/1 -> ri_to_c12/2
  a0_ch0/1 -> c_to_ri/1
  a0_ch1/1 -> c_to_ri1/1
  a0_ch2/1 -> c_to_ri2/1
  a0_ch3/1 -> c_to_ri3/1
  a1_ch0/1 -> c_to_ri4/1
  a1_ch1/1 -> c_to_ri5/1
  a1_ch2/1 -> c_to_ri6/1
  a1_ch3/1 -> c_to_ri7/1
  a2_ch0/1 -> c_to_ri8/1
  a2_ch1/1 -> c_to_ri9/1
  a2_ch2/1 -> c_to_ri10/1
  a2_ch3/1 -> c_to_ri11/1
  ri_to_c3/1 -> c0_ch0/1
  ri_to_c1/1 -> c0_ch1/1
  ri_to_c9/1 -> c0_ch2/1
  ri_to_c7/1 -> c0_ch3/1
  ri_to_c4/1 -> cx_ch0/1
  ri_to_c2/1 -> cx_ch1/1
  ri_to_c10/1 -> cx_ch2/1
  ri_to_c8/1 -> cx_ch3/1
  ri_to_c5/1 -> cy_ch0/1
  ri_to_c6/1 -> cy_ch1/1
  ri_to_c11/1 -> cy_ch2/1
  ri_to_c12/1 -> cy_ch3/1

== system doa_no_gotos/pipeline1 ==
  d : Inport
  Register{0..8} (9 alike) : xbsIndex_r4/Register  init=0  rst=off  en=off  dbl_ovrd=off  block_type=register
      Register0 settings: block_version=11.4
      Register1 settings: block_version=11.4
  q : Outport
  wires:
  Register0/1 -> Register1/1
  Register1/1 -> Register2/1
  Register2/1 -> Register3/1
  Register3/1 -> Register4/1
  Register4/1 -> Register5/1
  Register5/1 -> Register6/1
  Register6/1 -> Register7/1
  Register7/1 -> Register8/1
  d/1 -> Register0/1
  Register8/1 -> q/1

== system doa_no_gotos/pipeline5 ==
  d : Inport
  Register{0..8} (9 alike) : xbsIndex_r4/Register  init=0  rst=off  en=off  dbl_ovrd=off  block_type=register
      Register0 settings: block_version=11.4
      Register1 settings: block_version=11.4
  q : Outport
  wires:
  Register0/1 -> Register1/1
  Register1/1 -> Register2/1
  Register2/1 -> Register3/1
  Register3/1 -> Register4/1
  Register4/1 -> Register5/1
  Register5/1 -> Register6/1
  Register6/1 -> Register7/1
  Register7/1 -> Register8/1
  d/1 -> Register0/1
  Register8/1 -> q/1

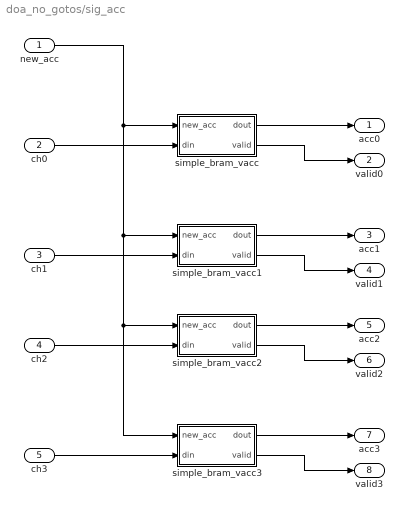
== system doa_no_gotos/sig_acc ==
  new_acc : Inport
  ch0 : Inport  Port=2
  ch1 : Inport  Port=3
  ch2 : Inport  Port=4
  ch3 : Inport  Port=5
  simple_bram_vacc : Subsystem  AncestorBlock=casper_library_accumulators/simple_bram_vacc  mask(simple_bram_vacc){vec_len=512, arith_type=Signed, n_bits=32, bin_pt=0}
      mask prompts: vec_len "Vector length:"; arith_type "Output type:"; n_bits "Bit width (output):"; bin_pt "Binary point (output):"
      mask help: This simple vector accumulator is based on a shift register. It outputs its previous accumulated vector after a new_acc pulse is received.
      mask init:
      | simple_bram_vacc_init(gcb, ...
      |     'vec_len', vec_len, ...
      |     'arith_type', arith_type, ...
      |     'n_bits', n_bits, ...
      |     'bin_pt', bin_pt);
      mask TypeOptions arith_type: Signed | Unsigned
  simple_bram_vacc1 : Subsystem  AncestorBlock=casper_library_accumulators/simple_bram_vacc  mask(simple_bram_vacc){vec_len=512, arith_type=Signed, n_bits=32, bin_pt=0}
      mask prompts: vec_len "Vector length:"; arith_type "Output type:"; n_bits "Bit width (output):"; bin_pt "Binary point (output):"
      mask help: This simple vector accumulator is based on a shift register. It outputs its previous accumulated vector after a new_acc pulse is received.
      mask init:
      | simple_bram_vacc_init(gcb, ...
      |     'vec_len', vec_len, ...
      |     'arith_type', arith_type, ...
      |     'n_bits', n_bits, ...
      |     'bin_pt', bin_pt);
      mask TypeOptions arith_type: Signed | Unsigned
  simple_bram_vacc2 : Subsystem  AncestorBlock=casper_library_accumulators/simple_bram_vacc  mask(simple_bram_vacc){vec_len=512, arith_type=Signed, n_bits=32, bin_pt=0}
      mask prompts: vec_len "Vector length:"; arith_type "Output type:"; n_bits "Bit width (output):"; bin_pt "Binary point (output):"
      mask help: This simple vector accumulator is based on a shift register. It outputs its previous accumulated vector after a new_acc pulse is received.
      mask init:
      | simple_bram_vacc_init(gcb, ...
      |     'vec_len', vec_len, ...
      |     'arith_type', arith_type, ...
      |     'n_bits', n_bits, ...
      |     'bin_pt', bin_pt);
      mask TypeOptions arith_type: Signed | Unsigned
  simple_bram_vacc3 : Subsystem  AncestorBlock=casper_library_accumulators/simple_bram_vacc  mask(simple_bram_vacc){vec_len=512, arith_type=Signed, n_bits=32, bin_pt=0}
      mask prompts: vec_len "Vector length:"; arith_type "Output type:"; n_bits "Bit width (output):"; bin_pt "Binary point (output):"
      mask help: This simple vector accumulator is based on a shift register. It outputs its previous accumulated vector after a new_acc pulse is received.
      mask init:
      | simple_bram_vacc_init(gcb, ...
      |     'vec_len', vec_len, ...
      |     'arith_type', arith_type, ...
      |     'n_bits', n_bits, ...
      |     'bin_pt', bin_pt);
      mask TypeOptions arith_type: Signed | Unsigned
  acc0 : Outport
  valid0 : Outport  Port=2
  acc1 : Outport  Port=3
  valid1 : Outport  Port=4
  acc2 : Outport  Port=5
  valid2 : Outport  Port=6
  acc3 : Outport  Port=7
  valid3 : Outport  Port=8
  wires:
  simple_bram_vacc/1(dout) -> acc0/1
  simple_bram_vacc/2(valid) -> valid0/1
  ch0/1 -> simple_bram_vacc/2(din)
  simple_bram_vacc1/1(dout) -> acc1/1
  simple_bram_vacc1/2(valid) -> valid1/1
  ch1/1 -> simple_bram_vacc1/2(din)
  simple_bram_vacc2/2(valid) -> valid2/1
  new_acc/1 -> simple_bram_vacc2/1(new_acc), simple_bram_vacc3/1(new_acc), simple_bram_vacc1/1(new_acc), simple_bram_vacc/1(new_acc)
  ch2/1 -> simple_bram_vacc2/2(din)
  simple_bram_vacc3/1(dout) -> acc3/1
  simple_bram_vacc3/2(valid) -> valid3/1
  ch3/1 -> simple_bram_vacc3/2(din)
  simple_bram_vacc2/1(dout) -> acc2/1

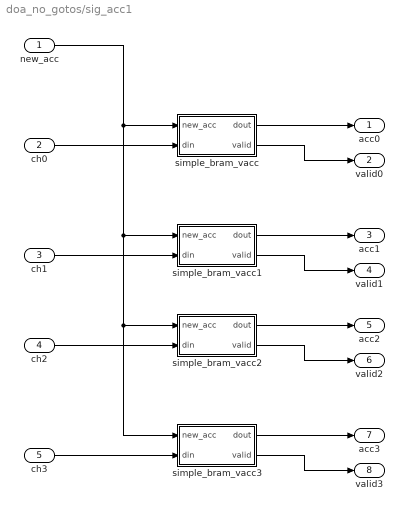
== system doa_no_gotos/sig_acc1 ==
  new_acc : Inport
  ch0 : Inport  Port=2
  ch1 : Inport  Port=3
  ch2 : Inport  Port=4
  ch3 : Inport  Port=5
  simple_bram_vacc : Subsystem  AncestorBlock=casper_library_accumulators/simple_bram_vacc  mask(simple_bram_vacc){vec_len=512, arith_type=Signed, n_bits=32, bin_pt=0}
      mask prompts: vec_len "Vector length:"; arith_type "Output type:"; n_bits "Bit width (output):"; bin_pt "Binary point (output):"
      mask help: This simple vector accumulator is based on a shift register. It outputs its previous accumulated vector after a new_acc pulse is received.
      mask init:
      | simple_bram_vacc_init(gcb, ...
      |     'vec_len', vec_len, ...
      |     'arith_type', arith_type, ...
      |     'n_bits', n_bits, ...
      |     'bin_pt', bin_pt);
      mask TypeOptions arith_type: Signed | Unsigned
  simple_bram_vacc1 : Subsystem  AncestorBlock=casper_library_accumulators/simple_bram_vacc  mask(simple_bram_vacc){vec_len=512, arith_type=Signed, n_bits=32, bin_pt=0}
      mask prompts: vec_len "Vector length:"; arith_type "Output type:"; n_bits "Bit width (output):"; bin_pt "Binary point (output):"
      mask help: This simple vector accumulator is based on a shift register. It outputs its previous accumulated vector after a new_acc pulse is received.
      mask init:
      | simple_bram_vacc_init(gcb, ...
      |     'vec_len', vec_len, ...
      |     'arith_type', arith_type, ...
      |     'n_bits', n_bits, ...
      |     'bin_pt', bin_pt);
      mask TypeOptions arith_type: Signed | Unsigned
  simple_bram_vacc2 : Subsystem  AncestorBlock=casper_library_accumulators/simple_bram_vacc  mask(simple_bram_vacc){vec_len=512, arith_type=Signed, n_bits=32, bin_pt=0}
      mask prompts: vec_len "Vector length:"; arith_type "Output type:"; n_bits "Bit width (output):"; bin_pt "Binary point (output):"
      mask help: This simple vector accumulator is based on a shift register. It outputs its previous accumulated vector after a new_acc pulse is received.
      mask init:
      | simple_bram_vacc_init(gcb, ...
      |     'vec_len', vec_len, ...
      |     'arith_type', arith_type, ...
      |     'n_bits', n_bits, ...
      |     'bin_pt', bin_pt);
      mask TypeOptions arith_type: Signed | Unsigned
  simple_bram_vacc3 : Subsystem  AncestorBlock=casper_library_accumulators/simple_bram_vacc  mask(simple_bram_vacc){vec_len=512, arith_type=Signed, n_bits=32, bin_pt=0}
      mask prompts: vec_len "Vector length:"; arith_type "Output type:"; n_bits "Bit width (output):"; bin_pt "Binary point (output):"
      mask help: This simple vector accumulator is based on a shift register. It outputs its previous accumulated vector after a new_acc pulse is received.
      mask init:
      | simple_bram_vacc_init(gcb, ...
      |     'vec_len', vec_len, ...
      |     'arith_type', arith_type, ...
      |     'n_bits', n_bits, ...
      |     'bin_pt', bin_pt);
      mask TypeOptions arith_type: Signed | Unsigned
  acc0 : Outport
  valid0 : Outport  Port=2
  acc1 : Outport  Port=3
  valid1 : Outport  Port=4
  acc2 : Outport  Port=5
  valid2 : Outport  Port=6
  acc3 : Outport  Port=7
  valid3 : Outport  Port=8
  wires:
  simple_bram_vacc/1(dout) -> acc0/1
  simple_bram_vacc/2(valid) -> valid0/1
  ch0/1 -> simple_bram_vacc/2(din)
  simple_bram_vacc1/1(dout) -> acc1/1
  simple_bram_vacc1/2(valid) -> valid1/1
  ch1/1 -> simple_bram_vacc1/2(din)
  simple_bram_vacc2/2(valid) -> valid2/1
  new_acc/1 -> simple_bram_vacc2/1(new_acc), simple_bram_vacc3/1(new_acc), simple_bram_vacc1/1(new_acc), simple_bram_vacc/1(new_acc)
  ch2/1 -> simple_bram_vacc2/2(din)
  simple_bram_vacc3/1(dout) -> acc3/1
  simple_bram_vacc3/2(valid) -> valid3/1
  ch3/1 -> simple_bram_vacc3/2(din)
  simple_bram_vacc2/1(dout) -> acc2/1

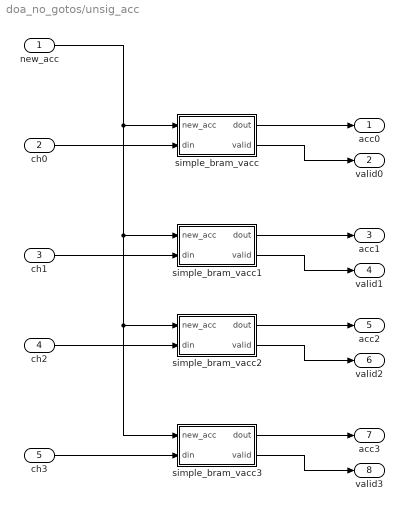
== system doa_no_gotos/unsig_acc ==
  new_acc : Inport
  ch0 : Inport  Port=2
  ch1 : Inport  Port=3
  ch2 : Inport  Port=4
  ch3 : Inport  Port=5
  simple_bram_vacc : Subsystem  AncestorBlock=casper_library_accumulators/simple_bram_vacc  mask(simple_bram_vacc){vec_len=512, arith_type=Unsigned, n_bits=32, bin_pt=0}
      mask prompts: vec_len "Vector length:"; arith_type "Output type:"; n_bits "Bit width (output):"; bin_pt "Binary point (output):"
      mask help: This simple vector accumulator is based on a shift register. It outputs its previous accumulated vector after a new_acc pulse is received.
      mask init:
      | simple_bram_vacc_init(gcb, ...
      |     'vec_len', vec_len, ...
      |     'arith_type', arith_type, ...
      |     'n_bits', n_bits, ...
      |     'bin_pt', bin_pt);
      mask TypeOptions arith_type: Signed | Unsigned
  simple_bram_vacc1 : Subsystem  AncestorBlock=casper_library_accumulators/simple_bram_vacc  mask(simple_bram_vacc){vec_len=512, arith_type=Unsigned, n_bits=32, bin_pt=0}
      mask prompts: vec_len "Vector length:"; arith_type "Output type:"; n_bits "Bit width (output):"; bin_pt "Binary point (output):"
      mask help: This simple vector accumulator is based on a shift register. It outputs its previous accumulated vector after a new_acc pulse is received.
      mask init:
      | simple_bram_vacc_init(gcb, ...
      |     'vec_len', vec_len, ...
      |     'arith_type', arith_type, ...
      |     'n_bits', n_bits, ...
      |     'bin_pt', bin_pt);
      mask TypeOptions arith_type: Signed | Unsigned
  simple_bram_vacc2 : Subsystem  AncestorBlock=casper_library_accumulators/simple_bram_vacc  mask(simple_bram_vacc){vec_len=512, arith_type=Unsigned, n_bits=32, bin_pt=0}
      mask prompts: vec_len "Vector length:"; arith_type "Output type:"; n_bits "Bit width (output):"; bin_pt "Binary point (output):"
      mask help: This simple vector accumulator is based on a shift register. It outputs its previous accumulated vector after a new_acc pulse is received.
      mask init:
      | simple_bram_vacc_init(gcb, ...
      |     'vec_len', vec_len, ...
      |     'arith_type', arith_type, ...
      |     'n_bits', n_bits, ...
      |     'bin_pt', bin_pt);
      mask TypeOptions arith_type: Signed | Unsigned
  simple_bram_vacc3 : Subsystem  AncestorBlock=casper_library_accumulators/simple_bram_vacc  mask(simple_bram_vacc){vec_len=512, arith_type=Unsigned, n_bits=32, bin_pt=0}
      mask prompts: vec_len "Vector length:"; arith_type "Output type:"; n_bits "Bit width (output):"; bin_pt "Binary point (output):"
      mask help: This simple vector accumulator is based on a shift register. It outputs its previous accumulated vector after a new_acc pulse is received.
      mask init:
      | simple_bram_vacc_init(gcb, ...
      |     'vec_len', vec_len, ...
      |     'arith_type', arith_type, ...
      |     'n_bits', n_bits, ...
      |     'bin_pt', bin_pt);
      mask TypeOptions arith_type: Signed | Unsigned
  acc0 : Outport
  valid0 : Outport  Port=2
  acc1 : Outport  Port=3
  valid1 : Outport  Port=4
  acc2 : Outport  Port=5
  valid2 : Outport  Port=6
  acc3 : Outport  Port=7
  valid3 : Outport  Port=8
  wires:
  simple_bram_vacc/1(dout) -> acc0/1
  simple_bram_vacc/2(valid) -> valid0/1
  ch0/1 -> simple_bram_vacc/2(din)
  simple_bram_vacc1/1(dout) -> acc1/1
  simple_bram_vacc1/2(valid) -> valid1/1
  ch1/1 -> simple_bram_vacc1/2(din)
  simple_bram_vacc2/2(valid) -> valid2/1
  new_acc/1 -> simple_bram_vacc3/1(new_acc), simple_bram_vacc2/1(new_acc), simple_bram_vacc1/1(new_acc), simple_bram_vacc/1(new_acc)
  ch2/1 -> simple_bram_vacc2/2(din)
  simple_bram_vacc3/1(dout) -> acc3/1
  simple_bram_vacc3/2(valid) -> valid3/1
  ch3/1 -> simple_bram_vacc3/2(din)
  simple_bram_vacc2/1(dout) -> acc2/1
